simulink model "LFC_PID"  (Simulink 7.8)
settings: Solver=ode8  StartTime=0.0  StopTime=60  FixedStep=0.01  RelTol=1e-3
values from neighbouring files (symbols this model uses):
  DPd1 = In(2)    [AREA1.m]    (also in Main.m = 0.3)
  DPd2 = In(2)    [AREA2.m]    (also in Main.m = 0.1)
  DPd3 = In(2)    [AREA3.m]    (also in Main.m = 0.01)
libraries: simulink x3
settings Model: Creator=Mahdi  LastModifiedBy=Mahdi

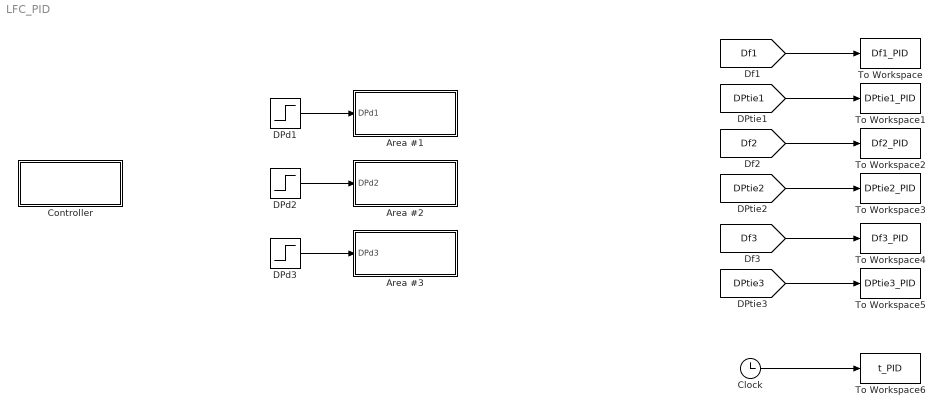
== system LFC_PID ==
  Area #1 : Subsystem
  Area #2 : Subsystem
  Area #3 : Subsystem
  Clock : Clock
  Controller : Subsystem
  DPd1 : Step  Time=0  After=DPd1  SampleTime=0
  DPd2 : Step  Time=0  After=DPd2  SampleTime=0
  DPd3 : Step  Time=0  After=DPd3  SampleTime=0
  To Workspace : ToWorkspace  VariableName=Df1_PID  SampleTime=-1  SaveFormat=Array
  To Workspace1 : ToWorkspace  VariableName=DPtie1_PID  SampleTime=-1  SaveFormat=Array
  To Workspace2 : ToWorkspace  VariableName=Df2_PID  SampleTime=-1  SaveFormat=Array
  To Workspace3 : ToWorkspace  VariableName=DPtie2_PID  SampleTime=-1  SaveFormat=Array
  To Workspace4 : ToWorkspace  VariableName=Df3_PID  SampleTime=-1  SaveFormat=Array
  To Workspace5 : ToWorkspace  VariableName=DPtie3_PID  SampleTime=-1  SaveFormat=Array
  To Workspace6 : ToWorkspace  VariableName=t_PID  SampleTime=-1  SaveFormat=Array
  wires:
  DPd1/1 -> Area #1/1(DPd1)
  DPd2/1 -> Area #2/1(DPd2)
  DPd3/1 -> Area #3/1(DPd3)
  [Df1] -> To Workspace/1
  [DPtie1] -> To Workspace1/1
  [Df2] -> To Workspace2/1
  [DPtie2] -> To Workspace3/1
  [Df3] -> To Workspace4/1
  [DPtie3] -> To Workspace5/1
  Clock/1 -> To Workspace6/1

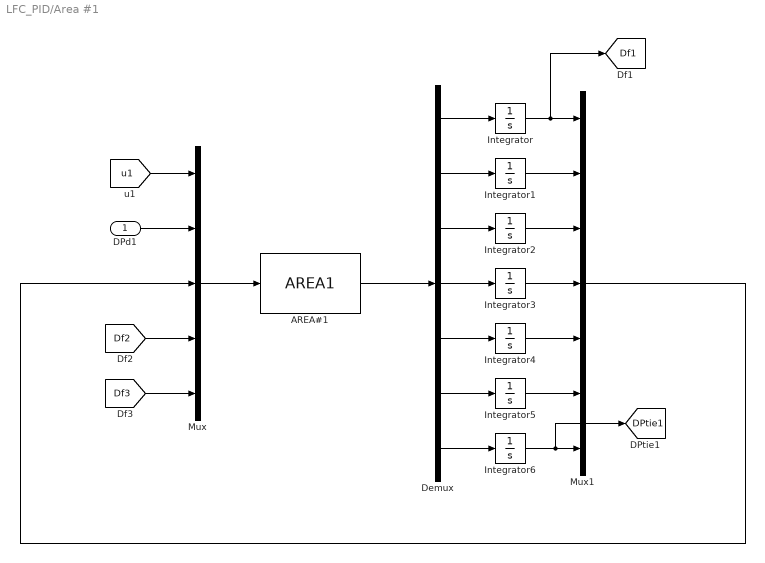
== system LFC_PID/Area #1 ==
  DPd1 : Inport
  AREA#1 : MATLABFcn  MATLABFcn=AREA1
  Demux : Demux  Outputs=7
  Integrator{,1..6} (7 alike) : Integrator
  Mux : Mux  Inputs=5
  Mux1 : Mux  Inputs=7
  tag scope: DPtie1=global, Df1=global
  wires:
  AREA#1/1 -> Demux/1
  Mux/1 -> AREA#1/1
  Demux/1 -> Integrator/1
  Demux/2 -> Integrator1/1
  Demux/3 -> Integrator2/1
  Demux/4 -> Integrator3/1
  Demux/5 -> Integrator4/1
  Demux/6 -> Integrator5/1
  Demux/7 -> Integrator6/1
  Integrator/1 -> Mux1/1, [Df1]
  Integrator1/1 -> Mux1/2
  Integrator2/1 -> Mux1/3
  Integrator3/1 -> Mux1/4
  Integrator4/1 -> Mux1/5
  Integrator6/1 -> Mux1/7, [DPtie1]
  Integrator5/1 -> Mux1/6
  [u1] -> Mux/1
  DPd1/1 -> Mux/2
  [Df2] -> Mux/4
  [Df3] -> Mux/5
  Mux1/1 -> Mux/3

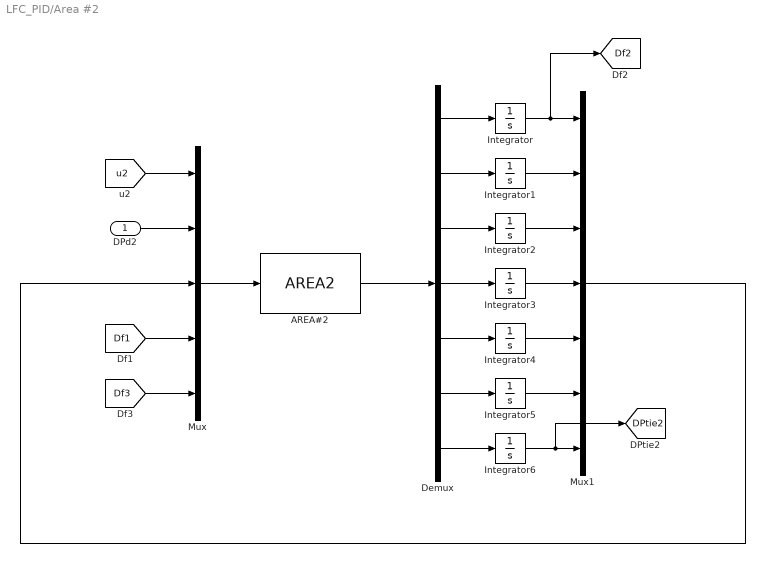
== system LFC_PID/Area #2 ==
  DPd2 : Inport
  AREA#2 : MATLABFcn  MATLABFcn=AREA2
  Demux : Demux  Outputs=7
  Integrator{,1..6} (7 alike) : Integrator
  Mux : Mux  Inputs=5
  Mux1 : Mux  Inputs=7
  tag scope: DPtie2=global, Df2=global
  wires:
  AREA#2/1 -> Demux/1
  Mux/1 -> AREA#2/1
  Demux/1 -> Integrator/1
  Demux/2 -> Integrator1/1
  Demux/3 -> Integrator2/1
  Demux/4 -> Integrator3/1
  Demux/5 -> Integrator4/1
  Demux/6 -> Integrator5/1
  Demux/7 -> Integrator6/1
  Integrator/1 -> Mux1/1, [Df2]
  Integrator1/1 -> Mux1/2
  Integrator2/1 -> Mux1/3
  Integrator3/1 -> Mux1/4
  Integrator4/1 -> Mux1/5
  Integrator6/1 -> Mux1/7, [DPtie2]
  Integrator5/1 -> Mux1/6
  Mux1/1 -> Mux/3
  [u2] -> Mux/1
  DPd2/1 -> Mux/2
  [Df1] -> Mux/4
  [Df3] -> Mux/5

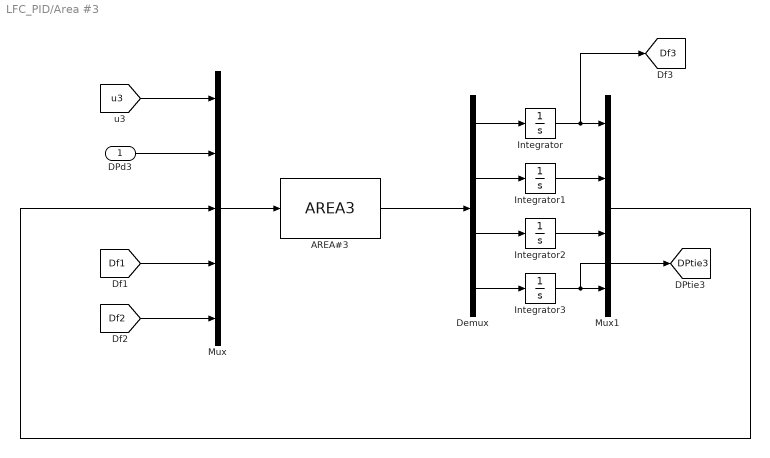
== system LFC_PID/Area #3 ==
  DPd3 : Inport
  AREA#3 : MATLABFcn  MATLABFcn=AREA3
  Demux : Demux
  Integrator{,1..3} (4 alike) : Integrator
  Mux : Mux  Inputs=5
  Mux1 : Mux
  tag scope: DPtie3=global, Df3=global
  wires:
  Demux/1 -> Integrator/1
  Demux/2 -> Integrator1/1
  Demux/3 -> Integrator2/1
  Demux/4 -> Integrator3/1
  Integrator/1 -> Mux1/1, [Df3]
  Integrator1/1 -> Mux1/2
  Integrator2/1 -> Mux1/3
  Integrator3/1 -> Mux1/4, [DPtie3]
  AREA#3/1 -> Demux/1
  Mux/1 -> AREA#3/1
  [u3] -> Mux/1
  DPd3/1 -> Mux/2
  [Df1] -> Mux/4
  [Df2] -> Mux/5
  Mux1/1 -> Mux/3

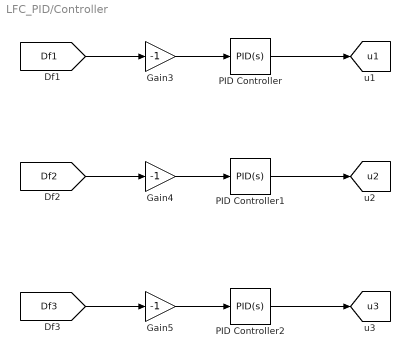
== system LFC_PID/Controller ==
  Gain3 : Gain  Gain=-1
  Gain4 : Gain  Gain=-1
  Gain5 : Gain  Gain=-1
  PID Controller : simulink/Continuous/PID Controller  Controller=PID  TimeDomain=Continuous-time  SampleTime=1  IntegratorMethod=Forward Euler  FilterMethod=Forward Euler  Form=Parallel  P=64.8  I=5.02  D=62.7  N=100  InitialConditionSource=internal  InitialConditionForIntegrator=0  InitialConditionForFilter=0  ExternalReset=none  LimitOutput=off  UpperSaturationLimit=inf  LowerSaturationLimit=-inf  LinearizeAsGain=off  AntiWindupMode=none  Kb=1  TrackingMode=off  Kt=1  PParamMin=[]  PParamMax=[]  IParamMin=[]  IParamMax=[]  DParamMin=[]  DParamMax=[]  NParamMin=[]  NParamMax=[]  KbParamMin=[]  KbParamMax=[]  KtParamMin=[]  KtParamMax=[]  POutMin=[]  POutMax=[]  IOutMin=[]  IOutMax=[]  DOutMin=[]  DOutMax=[]  NOutMin=[]  NOutMax=[]  KbOutMin=[]  KbOutMax=[]  KtOutMin=[]  KtOutMax=[]  IntegratorOutMin=[]  IntegratorOutMax=[]  FilterOutMin=[]  FilterOutMax=[]  SumOutMin=[]  SumOutMax=[]  SumI1OutMin=[]  SumI1OutMax=[]  SumI2OutMin=[]  SumI2OutMax=[]  SumI3OutMin=[]  SumI3OutMax=[]  SumDOutMin=[]  SumDOutMax=[]  SaturationOutMin=[]  SaturationOutMax=[]  IntegratorContinuousStateAttributes=''  IntegratorStateMustResolveToSignalObject=off  IntegratorRTWStateStorageClass=Auto  FilterContinuousStateAttributes=''  FilterStateMustResolveToSignalObject=off  FilterRTWStateStorageClass=Auto
  PID Controller1 : simulink/Continuous/PID Controller  Controller=PID  TimeDomain=Continuous-time  SampleTime=1  IntegratorMethod=Forward Euler  FilterMethod=Forward Euler  Form=Parallel  P=0.36  I=0.011  D=4.5  N=100  InitialConditionSource=internal  InitialConditionForIntegrator=0  InitialConditionForFilter=0  ExternalReset=none  LimitOutput=off  UpperSaturationLimit=inf  LowerSaturationLimit=-inf  LinearizeAsGain=off  AntiWindupMode=none  Kb=1  TrackingMode=off  Kt=1  PParamMin=[]  PParamMax=[]  IParamMin=[]  IParamMax=[]  DParamMin=[]  DParamMax=[]  NParamMin=[]  NParamMax=[]  KbParamMin=[]  KbParamMax=[]  KtParamMin=[]  KtParamMax=[]  POutMin=[]  POutMax=[]  IOutMin=[]  IOutMax=[]  DOutMin=[]  DOutMax=[]  NOutMin=[]  NOutMax=[]  KbOutMin=[]  KbOutMax=[]  KtOutMin=[]  KtOutMax=[]  IntegratorOutMin=[]  IntegratorOutMax=[]  FilterOutMin=[]  FilterOutMax=[]  SumOutMin=[]  SumOutMax=[]  SumI1OutMin=[]  SumI1OutMax=[]  SumI2OutMin=[]  SumI2OutMax=[]  SumI3OutMin=[]  SumI3OutMax=[]  SumDOutMin=[]  SumDOutMax=[]  SaturationOutMin=[]  SaturationOutMax=[]  IntegratorContinuousStateAttributes=''  IntegratorStateMustResolveToSignalObject=off  IntegratorRTWStateStorageClass=Auto  FilterContinuousStateAttributes=''  FilterStateMustResolveToSignalObject=off  FilterRTWStateStorageClass=Auto
  PID Controller2 : simulink/Continuous/PID Controller  Controller=PID  TimeDomain=Continuous-time  SampleTime=1  IntegratorMethod=Forward Euler  FilterMethod=Forward Euler  Form=Parallel  P=0.8  I=5.02  D=0.006  N=100  InitialConditionSource=internal  InitialConditionForIntegrator=0  InitialConditionForFilter=0  ExternalReset=none  LimitOutput=off  UpperSaturationLimit=inf  LowerSaturationLimit=-inf  LinearizeAsGain=off  AntiWindupMode=none  Kb=1  TrackingMode=off  Kt=1  PParamMin=[]  PParamMax=[]  IParamMin=[]  IParamMax=[]  DParamMin=[]  DParamMax=[]  NParamMin=[]  NParamMax=[]  KbParamMin=[]  KbParamMax=[]  KtParamMin=[]  KtParamMax=[]  POutMin=[]  POutMax=[]  IOutMin=[]  IOutMax=[]  DOutMin=[]  DOutMax=[]  NOutMin=[]  NOutMax=[]  KbOutMin=[]  KbOutMax=[]  KtOutMin=[]  KtOutMax=[]  IntegratorOutMin=[]  IntegratorOutMax=[]  FilterOutMin=[]  FilterOutMax=[]  SumOutMin=[]  SumOutMax=[]  SumI1OutMin=[]  SumI1OutMax=[]  SumI2OutMin=[]  SumI2OutMax=[]  SumI3OutMin=[]  SumI3OutMax=[]  SumDOutMin=[]  SumDOutMax=[]  SaturationOutMin=[]  SaturationOutMax=[]  IntegratorContinuousStateAttributes=''  IntegratorStateMustResolveToSignalObject=off  IntegratorRTWStateStorageClass=Auto  FilterContinuousStateAttributes=''  FilterStateMustResolveToSignalObject=off  FilterRTWStateStorageClass=Auto
  tag scope: u1=global, u2=global, u3=global
  wires:
  [Df1] -> Gain3/1
  [Df2] -> Gain4/1
  [Df3] -> Gain5/1
  PID Controller1/1 -> [u2]
  PID Controller2/1 -> [u3]
  PID Controller/1 -> [u1]
  Gain3/1 -> PID Controller/1
  Gain4/1 -> PID Controller1/1
  Gain5/1 -> PID Controller2/1
